simulink model "Lab5"  (R2023b)
settings: Solver=VariableStepAuto  StartTime=0.0  StopTime=10.0  RelTol=1e-3
undefined symbols (not defined in the file): Cf, K, Kd, Kf, Ki, Kp, Md, xe_initial
settings Model: Creator=chris  LastModifiedBy=chris

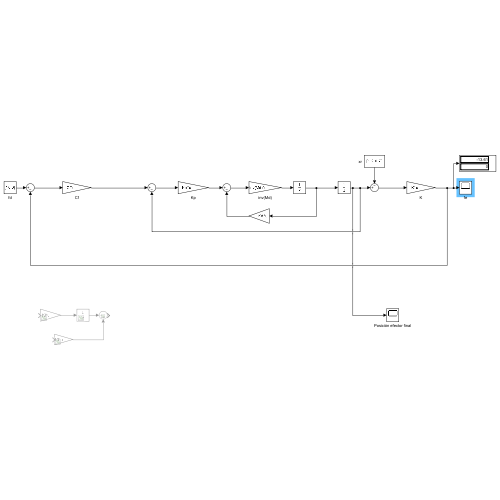
[thumbnail: Simulink's stored preview of the top-level diagram]
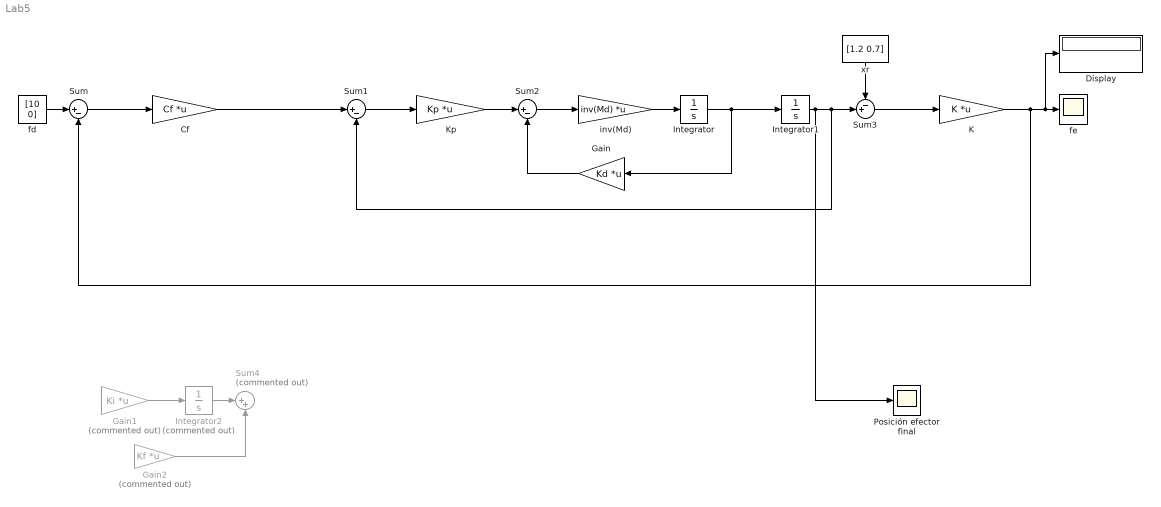
== system Lab5 ==
  Cf : Gain  Gain=Cf  Multiplication=Matrix(K*u)
  Display : Display
  Gain : Gain  Gain=Kd  Multiplication=Matrix(K*u)
  Gain1 : Gain  Commented=on  Gain=Ki  Multiplication=Matrix(K*u)
  Gain2 : Gain  Commented=on  Gain=Kf  Multiplication=Matrix(K*u)
  Integrator : Integrator  InitialCondition=xe_initial
  Integrator1 : Integrator  InitialCondition=xe_initial
  Integrator2 : Integrator  Commented=on  InitialCondition=xe_initial
  K : Gain  Gain=K  Multiplication=Matrix(K*u)
  Kp : Gain  Gain=Kp  Multiplication=Matrix(K*u)
  Posición efector final : Scope
  Sum : Sum  Inputs=|+-
  Sum1 : Sum  Inputs=|+-
  Sum2 : Sum  Inputs=|+-
  Sum3 : Sum  Inputs=-+|
  Sum4 : Sum  Commented=on  Inputs=|++
  fd : Constant  Value=[10 0]
  fe : Scope
  inv(Md) : Gain  Gain=inv(Md)  Multiplication=Matrix(K*u)
  xr : Constant  Value=[1.2 0.7]
  wires:
  fd/1 -> Sum/1
  Sum1/1 -> Kp/1
  Kp/1 -> Sum2/1
  Sum2/1 -> inv(Md)/1
  inv(Md)/1 -> Integrator/1
  Integrator/1 -> Gain/1, Integrator1/1
  K/1 -> Sum/2, Display/1, fe/1
  Integrator1/1 -> Posición efector final/1, Sum1/2, Sum3/2
  xr/1 -> Sum3/1
  Sum3/1 -> K/1
  Gain/1 -> Sum2/2
  Gain1/1 -> Integrator2/1
  Integrator2/1 -> Sum4/1
  Gain2/1 -> Sum4/2
  Sum/1 -> Cf/1
  Cf/1 -> Sum1/1
